simulink model "Mooventure2016_Rev5"  (Simulink 7.7)
settings: Solver=FixedStepDiscrete  StartTime=0.0  StopTime=10  RelTol=1e-3
PreLoadFcn:
  | try, eval([bdroot '_setup']); catch, eval('model_setup', ''); end
InitFcn:
  | try, eval([bdroot '_setup']); catch, eval('model_setup', ''); end
undefined symbols (not defined in the file): ECM, H1, motohawk_build_version, motohawk_trunc_name, motohawk_vardec_config_group, motohawk_vardec_path, xD
libraries: MotoHawk_lib x976, motohawk_control_primitives_lib x41, simulink x27, motohawk_annotations_lib x3
(part 3 of 16)

== system Mooventure2016_Rev5/Foreground/Inputs/ABS ==
  Bus Creator : BusCreator
  Bus Creator1 : BusCreator  Inputs=5
  Bus Creator2 : BusCreator  Inputs=2
  Bus Creator3 : BusCreator  Inputs=3
  Read CAN Message : MotoHawk_lib/CAN Blocks/Read CAN Message  nam=['CAN_' num2str(1)]  bus=-2  msg=CANRx_ABS_217  queue=1  slot=''  valid=off  stale=on  labelwires=on
  Read CAN Message1 : MotoHawk_lib/CAN Blocks/Read CAN Message  nam=['CAN_' num2str(1)]  bus=-2  msg=CANRx_ABS_4B0  queue=1  slot=''  valid=off  stale=on  labelwires=on
  Read CAN Message2 : MotoHawk_lib/CAN Blocks/Read CAN Message  nam=['CAN_' num2str(1)]  bus=-2  msg=CANRx_ABS_417  queue=1  slot=''  valid=off  stale=on  labelwires=on
  motohawk_override_abs1 : MotoHawk_lib/Calibration & Probing Blocks/motohawk_override_abs  SystemSampleTime=-1  parent_name='RT_Wheel_Rolling_Count_Ovr'  parent_val=0  show_more=off  name_source=Use Parameter  parent_read_level=1  parent_override_level=1  view_as=Number  enum_struct={'Disabled', 'Enabled'}  use_help_units=off  parent_help=''  parent_units=''  use_min_max=off  parent_min=-inf  parent_max=inf  use_precision=off  parent_precision=''  parent_gain=1  parent_offset=0  parent_exp=1  use_mototune_group=off  parent_group=motohawk_vardec_path(gcb)
  motohawk_override_abs10 : MotoHawk_lib/Calibration & Probing Blocks/motohawk_override_abs  SystemSampleTime=-1  parent_name='TCS_ENG_EVNT_IN_PROGRESS_Ovr'  parent_val=0  show_more=off  name_source=Use Parameter  parent_read_level=1  parent_override_level=1  view_as=Number  enum_struct={'Disabled', 'Enabled'}  use_help_units=off  parent_help=''  parent_units=''  use_min_max=off  parent_min=-inf  parent_max=inf  use_precision=off  parent_precision=''  parent_gain=1  parent_offset=0  parent_exp=1  use_mototune_group=off  parent_group=motohawk_vardec_path(gcb)
  motohawk_override_abs11 : MotoHawk_lib/Calibration & Probing Blocks/motohawk_override_abs  SystemSampleTime=-1  parent_name='ABS_417_AgeCount_Ovr'  parent_val=0  show_more=off  name_source=Use Parameter  parent_read_level=1  parent_override_level=1  view_as=Number  enum_struct={'Disabled', 'Enabled'}  use_help_units=off  parent_help=''  parent_units=''  use_min_max=off  parent_min=-inf  parent_max=inf  use_precision=off  parent_precision=''  parent_gain=1  parent_offset=0  parent_exp=1  use_mototune_group=off  parent_group=motohawk_vardec_path(gcb)
  motohawk_override_abs2 : MotoHawk_lib/Calibration & Probing Blocks/motohawk_override_abs  SystemSampleTime=-1  parent_name='Wheel_Rolling_Timestamp_Ovr'  parent_val=0  show_more=off  name_source=Use Parameter  parent_read_level=1  parent_override_level=1  view_as=Number  enum_struct={'Disabled', 'Enabled'}  use_help_units=off  parent_help=''  parent_units=''  use_min_max=off  parent_min=-inf  parent_max=inf  use_precision=off  parent_precision=''  parent_gain=1  parent_offset=0  parent_exp=1  use_mototune_group=off  parent_group=motohawk_vardec_path(gcb)
  motohawk_override_abs3 : MotoHawk_lib/Calibration & Probing Blocks/motohawk_override_abs  SystemSampleTime=-1  parent_name='ABS_217_AgeCount_Ovr'  parent_val=0  show_more=off  name_source=Use Parameter  parent_read_level=1  parent_override_level=1  view_as=Number  enum_struct={'Disabled', 'Enabled'}  use_help_units=off  parent_help=''  parent_units=''  use_min_max=off  parent_min=-inf  parent_max=inf  use_precision=off  parent_precision=''  parent_gain=1  parent_offset=0  parent_exp=1  use_mototune_group=off  parent_group=motohawk_vardec_path(gcb)
  motohawk_override_abs4 : MotoHawk_lib/Calibration & Probing Blocks/motohawk_override_abs  SystemSampleTime=-1  parent_name='Front_right_whl_speed_Ovr'  parent_val=0  show_more=off  name_source=Use Parameter  parent_read_level=1  parent_override_level=1  view_as=Number  enum_struct={'Disabled', 'Enabled'}  use_help_units=off  parent_help=''  parent_units=''  use_min_max=off  parent_min=-inf  parent_max=inf  use_precision=off  parent_precision=''  parent_gain=1  parent_offset=0  parent_exp=1  use_mototune_group=off  parent_group=motohawk_vardec_path(gcb)
  motohawk_override_abs5 : MotoHawk_lib/Calibration & Probing Blocks/motohawk_override_abs  SystemSampleTime=-1  parent_name='Rear_left_whl_speed_Ovr'  parent_val=0  show_more=off  name_source=Use Parameter  parent_read_level=1  parent_override_level=1  view_as=Number  enum_struct={'Disabled', 'Enabled'}  use_help_units=off  parent_help=''  parent_units=''  use_min_max=off  parent_min=-inf  parent_max=inf  use_precision=off  parent_precision=''  parent_gain=1  parent_offset=0  parent_exp=1  use_mototune_group=off  parent_group=motohawk_vardec_path(gcb)
  motohawk_override_abs6 : MotoHawk_lib/Calibration & Probing Blocks/motohawk_override_abs  SystemSampleTime=-1  parent_name='ABS_4B0_AgeCount_Ovr'  parent_val=0  show_more=off  name_source=Use Parameter  parent_read_level=1  parent_override_level=1  view_as=Number  enum_struct={'Disabled', 'Enabled'}  use_help_units=off  parent_help=''  parent_units=''  use_min_max=off  parent_min=-inf  parent_max=inf  use_precision=off  parent_precision=''  parent_gain=1  parent_offset=0  parent_exp=1  use_mototune_group=off  parent_group=motohawk_vardec_path(gcb)
  motohawk_override_abs7 : MotoHawk_lib/Calibration & Probing Blocks/motohawk_override_abs  SystemSampleTime=-1  parent_name='LF_Wheel_Rolling_Count_Ovr'  parent_val=0  show_more=off  name_source=Use Parameter  parent_read_level=1  parent_override_level=1  view_as=Number  enum_struct={'Disabled', 'Enabled'}  use_help_units=off  parent_help=''  parent_units=''  use_min_max=off  parent_min=-inf  parent_max=inf  use_precision=off  parent_precision=''  parent_gain=1  parent_offset=0  parent_exp=1  use_mototune_group=off  parent_group=motohawk_vardec_path(gcb)
  motohawk_override_abs8 : MotoHawk_lib/Calibration & Probing Blocks/motohawk_override_abs  SystemSampleTime=-1  parent_name='Front_left_whl_speed_Ovr'  parent_val=0  show_more=off  name_source=Use Parameter  parent_read_level=1  parent_override_level=1  view_as=Number  enum_struct={'Disabled', 'Enabled'}  use_help_units=off  parent_help=''  parent_units=''  use_min_max=off  parent_min=-inf  parent_max=inf  use_precision=off  parent_precision=''  parent_gain=1  parent_offset=0  parent_exp=1  use_mototune_group=off  parent_group=motohawk_vardec_path(gcb)
  motohawk_override_abs9 : MotoHawk_lib/Calibration & Probing Blocks/motohawk_override_abs  SystemSampleTime=-1  parent_name='Rear_right_whl_speed_Ovr'  parent_val=0  show_more=off  name_source=Use Parameter  parent_read_level=1  parent_override_level=1  view_as=Number  enum_struct={'Disabled', 'Enabled'}  use_help_units=off  parent_help=''  parent_units=''  use_min_max=off  parent_min=-inf  parent_max=inf  use_precision=off  parent_precision=''  parent_gain=1  parent_offset=0  parent_exp=1  use_mototune_group=off  parent_group=motohawk_vardec_path(gcb)
  motohawk_probe1 : MotoHawk_lib/Calibration & Probing Blocks/motohawk_probe  nam='RT_Wheel_Rolling_Count_Prb'  show_more=off  name_source=Use Parameter  read_level=1  view_as=Number  enum_struct={'Disabled', 'Enabled'}  vector_style=Wide Row  use_help_units=off  help=''  units=''  use_header_enum=off  row_header_enum={}  col_header_enum={}  use_precision=off  precision=''  gain=1  offset=0  exp=1  use_mototune_group=off  mototune_group=motohawk_vardec_path(gcb)
  motohawk_probe10 : MotoHawk_lib/Calibration & Probing Blocks/motohawk_probe  nam='TCS_ENG_EVNT_IN_PROGRESS_Prb'  show_more=off  name_source=Use Parameter  read_level=1  view_as=Number  enum_struct={'Disabled', 'Enabled'}  vector_style=Wide Row  use_help_units=off  help=''  units=''  use_header_enum=off  row_header_enum={}  col_header_enum={}  use_precision=off  precision=''  gain=1  offset=0  exp=1  use_mototune_group=off  mototune_group=motohawk_vardec_path(gcb)
  motohawk_probe11 : MotoHawk_lib/Calibration & Probing Blocks/motohawk_probe  nam='ABS_417_AgeCount_Prb'  show_more=off  name_source=Use Parameter  read_level=1  view_as=Number  enum_struct={'Disabled', 'Enabled'}  vector_style=Wide Row  use_help_units=off  help=''  units=''  use_header_enum=off  row_header_enum={}  col_header_enum={}  use_precision=off  precision=''  gain=1  offset=0  exp=1  use_mototune_group=off  mototune_group=motohawk_vardec_path(gcb)
  motohawk_probe2 : MotoHawk_lib/Calibration & Probing Blocks/motohawk_probe  nam='Wheel_Rolling_Timestamp_Prb'  show_more=off  name_source=Use Parameter  read_level=1  view_as=Number  enum_struct={'Disabled', 'Enabled'}  vector_style=Wide Row  use_help_units=off  help=''  units=''  use_header_enum=off  row_header_enum={}  col_header_enum={}  use_precision=off  precision=''  gain=1  offset=0  exp=1  use_mototune_group=off  mototune_group=motohawk_vardec_path(gcb)
  motohawk_probe3 : MotoHawk_lib/Calibration & Probing Blocks/motohawk_probe  nam='ABS_217_AgeCount_Prb'  show_more=off  name_source=Use Parameter  read_level=1  view_as=Number  enum_struct={'Disabled', 'Enabled'}  vector_style=Wide Row  use_help_units=off  help=''  units=''  use_header_enum=off  row_header_enum={}  col_header_enum={}  use_precision=off  precision=''  gain=1  offset=0  exp=1  use_mototune_group=off  mototune_group=motohawk_vardec_path(gcb)
  motohawk_probe4 : MotoHawk_lib/Calibration & Probing Blocks/motohawk_probe  nam='Front_right_whl_speed_Prb'  show_more=off  name_source=Use Parameter  read_level=1  view_as=Number  enum_struct={'Disabled', 'Enabled'}  vector_style=Wide Row  use_help_units=off  help=''  units=''  use_header_enum=off  row_header_enum={}  col_header_enum={}  use_precision=off  precision=''  gain=1  offset=0  exp=1  use_mototune_group=off  mototune_group=motohawk_vardec_path(gcb)
  motohawk_probe5 : MotoHawk_lib/Calibration & Probing Blocks/motohawk_probe  nam='Rear_left_whl_speed_Prb'  show_more=off  name_source=Use Parameter  read_level=1  view_as=Number  enum_struct={'Disabled', 'Enabled'}  vector_style=Wide Row  use_help_units=off  help=''  units=''  use_header_enum=off  row_header_enum={}  col_header_enum={}  use_precision=off  precision=''  gain=1  offset=0  exp=1  use_mototune_group=off  mototune_group=motohawk_vardec_path(gcb)
  motohawk_probe6 : MotoHawk_lib/Calibration & Probing Blocks/motohawk_probe  nam='ABS_4B0_AgeCount_Prb'  show_more=off  name_source=Use Parameter  read_level=1  view_as=Number  enum_struct={'Disabled', 'Enabled'}  vector_style=Wide Row  use_help_units=off  help=''  units=''  use_header_enum=off  row_header_enum={}  col_header_enum={}  use_precision=off  precision=''  gain=1  offset=0  exp=1  use_mototune_group=off  mototune_group=motohawk_vardec_path(gcb)
  motohawk_probe7 : MotoHawk_lib/Calibration & Probing Blocks/motohawk_probe  nam='LF_Wheel_Rolling_Count_Prb'  show_more=off  name_source=Use Parameter  read_level=1  view_as=Number  enum_struct={'Disabled', 'Enabled'}  vector_style=Wide Row  use_help_units=off  help=''  units=''  use_header_enum=off  row_header_enum={}  col_header_enum={}  use_precision=off  precision=''  gain=1  offset=0  exp=1  use_mototune_group=off  mototune_group=motohawk_vardec_path(gcb)
  motohawk_probe8 : MotoHawk_lib/Calibration & Probing Blocks/motohawk_probe  nam='Front_left_whl_speed_Prb'  show_more=off  name_source=Use Parameter  read_level=1  view_as=Number  enum_struct={'Disabled', 'Enabled'}  vector_style=Wide Row  use_help_units=off  help=''  units=''  use_header_enum=off  row_header_enum={}  col_header_enum={}  use_precision=off  precision=''  gain=1  offset=0  exp=1  use_mototune_group=off  mototune_group=motohawk_vardec_path(gcb)
  motohawk_probe9 : MotoHawk_lib/Calibration & Probing Blocks/motohawk_probe  nam='Rear_right_whl_speed_Prb'  show_more=off  name_source=Use Parameter  read_level=1  view_as=Number  enum_struct={'Disabled', 'Enabled'}  vector_style=Wide Row  use_help_units=off  help=''  units=''  use_header_enum=off  row_header_enum={}  col_header_enum={}  use_precision=off  precision=''  gain=1  offset=0  exp=1  use_mototune_group=off  mototune_group=motohawk_vardec_path(gcb)
  Out1 : Outport
  wires:
  Read CAN Message/1 -> motohawk_override_abs3/1, motohawk_probe3/1  "AgeCount"
  Read CAN Message/2 -> motohawk_override_abs7/1, motohawk_probe7/1  "LF_Wheel_Rolling_Count"
  Read CAN Message/3 -> motohawk_override_abs1/1, motohawk_probe1/1  "RT_Wheel_Rolling_Count"
  Read CAN Message/4 -> motohawk_override_abs2/1, motohawk_probe2/1  "Wheel_Rolling_Timestamp"
  motohawk_override_abs3/1 -> Bus Creator/1  "AgeCount 217"
  motohawk_override_abs7/1 -> Bus Creator/2  "LF Wheel Rolling Count"
  motohawk_override_abs1/1 -> Bus Creator/3  "RT Wheel Rolling Count"
  motohawk_override_abs2/1 -> Bus Creator/4  "Wheel Rolling Timestamp"
  Read CAN Message1/2 -> motohawk_override_abs8/1, motohawk_probe8/1  "Front_left_whl_speed"
  Read CAN Message1/3 -> motohawk_override_abs4/1, motohawk_probe4/1  "Front_right_whl_speed"
  Read CAN Message1/4 -> motohawk_override_abs5/1, motohawk_probe5/1  "Rear_left_whl_speed"
  motohawk_override_abs6/1 -> Bus Creator1/1  "AgeCount 4B0"
  motohawk_override_abs8/1 -> Bus Creator1/2  "Front left whl speed"
  motohawk_override_abs4/1 -> Bus Creator1/3  "Front right whl speed"
  motohawk_override_abs5/1 -> Bus Creator1/4  "Rear left whl speed"
  Read CAN Message1/1 -> motohawk_override_abs6/1, motohawk_probe6/1  "AgeCount"
  Read CAN Message1/5 -> motohawk_override_abs9/1, motohawk_probe9/1  "Rear_right_whl_speed"
  motohawk_override_abs9/1 -> Bus Creator1/5  "Rear right whl speed"
  Read CAN Message2/1 -> motohawk_override_abs11/1, motohawk_probe11/1  "AgeCount"
  Read CAN Message2/2 -> motohawk_override_abs10/1, motohawk_probe10/1  "TCS_ENG_EVNT_IN_PROGRESS"
  motohawk_override_abs10/1 -> Bus Creator2/2  "ECS Eng Evnt In Progress"
  motohawk_override_abs11/1 -> Bus Creator2/1  "ABS 417 AgeCount"
  Bus Creator/1 -> Bus Creator3/1  "Tone Ring"
  Bus Creator1/1 -> Bus Creator3/2  "Wheel Speed"
  Bus Creator2/1 -> Bus Creator3/3  "Traction Control"
  Bus Creator3/1 -> Out1/1

== system Mooventure2016_Rev5/Foreground/Inputs/Analog Inputs ==
  note: TODO
  Bus Creator : BusCreator  Inputs=3
  Contactors : Subsystem
  Coolant : Subsystem
  DCDC Converter : Subsystem
  Out1 : Outport
  wires:
  Bus Creator/1 -> Out1/1
  Coolant/1(Out1) -> Bus Creator/1  "Coolant"
  DCDC Converter/1(Out1) -> Bus Creator/2  "DCDC"
  Contactors/1(Out1) -> Bus Creator/3  "Contactors"

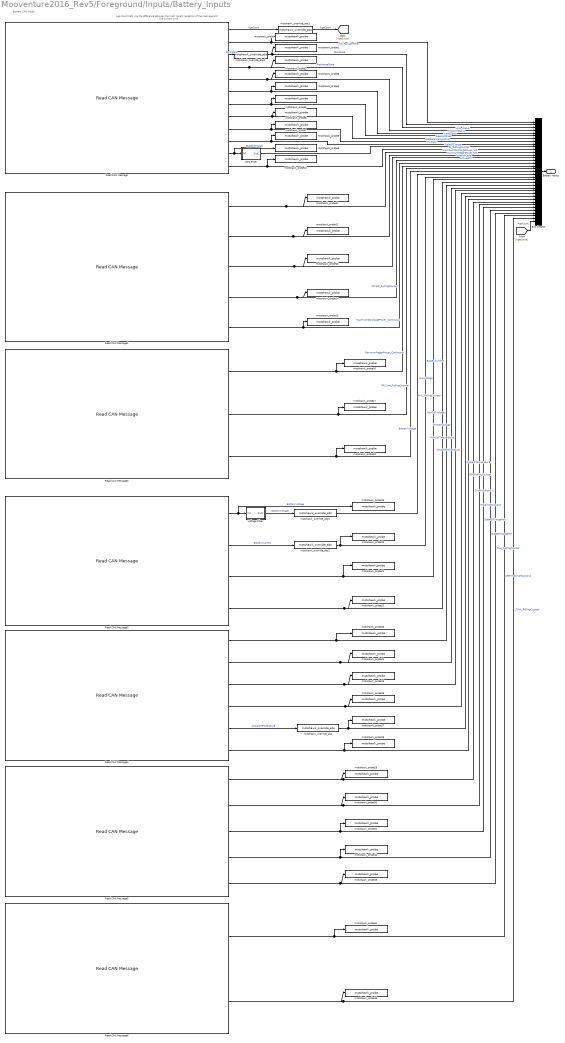
== system Mooventure2016_Rev5/Foreground/Inputs/Battery_Inputs ==
  note: Battery CAN inputs
  note: Age Count tells you the difference between the most recent reception of the message and the current time
  Bus Creator : BusCreator  Inputs=37
  Read CAN Message : MotoHawk_lib/CAN Blocks/Read CAN Message  nam=['CAN_' num2str(3)]  bus=-2  msg=CANRx_BATTERY_2FA  queue=1  slot=''  valid=off  stale=on  labelwires=on
  Read CAN Message1 : MotoHawk_lib/CAN Blocks/Read CAN Message  nam=['CAN_' num2str(3)]  bus=-2  msg=CANRx_BATTERY_2FB  queue=1  slot=''  valid=off  stale=off  labelwires=on
  Read CAN Message2 : MotoHawk_lib/CAN Blocks/Read CAN Message  nam=['CAN_' num2str(3)]  bus=-2  msg=CANRx_Battery_2FC  queue=1  slot=''  valid=off  stale=off  labelwires=on
  Read CAN Message3 : MotoHawk_lib/CAN Blocks/Read CAN Message  nam=['CAN_' num2str(3)]  bus=-2  msg=CANRx_Battery_2FD  queue=1  slot=''  valid=off  stale=off  labelwires=on
  Read CAN Message4 : MotoHawk_lib/CAN Blocks/Read CAN Message  nam=['CAN_' num2str(3)]  bus=-2  msg=CANRx_Battery_2FE  queue=1  slot=''  valid=off  stale=off  labelwires=on
  Read CAN Message5 : MotoHawk_lib/CAN Blocks/Read CAN Message  nam=['CAN_' num2str(3)]  bus=-2  msg=CANRx_Battery_2FF  queue=1  slot=''  valid=off  stale=off  labelwires=on
  Read CAN Message6 : MotoHawk_lib/CAN Blocks/Read CAN Message  nam=['CAN_' num2str(3)]  bus=-2  msg=CANRx_Battery_300  queue=1  slot=''  valid=off  stale=off  labelwires=on
  SOC Filter : Subsystem
  Voltage Filter : Subsystem
  motohawk_override_abs : MotoHawk_lib/Calibration & Probing Blocks/motohawk_override_abs  SystemSampleTime=-1  parent_name='Batt_Coolant_Temp_ovr'  parent_val=0  show_more=off  name_source=Use Parameter  parent_read_level=1  parent_override_level=1  view_as=Number  enum_struct={'Disabled', 'Enabled'}  use_help_units=off  parent_help=''  parent_units=''  use_min_max=off  parent_min=-inf  parent_max=inf  use_precision=off  parent_precision=''  parent_gain=1  parent_offset=0  parent_exp=1  use_mototune_group=off  parent_group=motohawk_vardec_path(gcb)
  motohawk_override_abs2 : MotoHawk_lib/Calibration & Probing Blocks/motohawk_override_abs  SystemSampleTime=-1  parent_name='Batt_Current_ovr'  parent_val=0  show_more=off  name_source=Use Parameter  parent_read_level=1  parent_override_level=1  view_as=Number  enum_struct={'Disabled', 'Enabled'}  use_help_units=off  parent_help=''  parent_units=''  use_min_max=off  parent_min=-inf  parent_max=inf  use_precision=off  parent_precision=''  parent_gain=1  parent_offset=0  parent_exp=1  use_mototune_group=off  parent_group=motohawk_vardec_path(gcb)
  motohawk_override_abs3 : MotoHawk_lib/Calibration & Probing Blocks/motohawk_override_abs  SystemSampleTime=-1  parent_name='Batt_Age_Count_ovr'  parent_val=0  show_more=off  name_source=Use Parameter  parent_read_level=1  parent_override_level=1  view_as=Number  enum_struct={'Disabled', 'Enabled'}  use_help_units=off  parent_help=''  parent_units=''  use_min_max=off  parent_min=-inf  parent_max=inf  use_precision=off  parent_precision=''  parent_gain=1  parent_offset=0  parent_exp=1  use_mototune_group=off  parent_group=motohawk_vardec_path(gcb)
  motohawk_override_abs4 : MotoHawk_lib/Calibration & Probing Blocks/motohawk_override_abs  SystemSampleTime=-1  parent_name='Pack_State_ovr'  parent_val=0  show_more=on  name_source=Use Parameter  parent_read_level=1  parent_override_level=1  view_as=Number  enum_struct={'Disabled', 'Enabled'}  use_help_units=off  parent_help=''  parent_units=''  use_min_max=on  parent_min=0  parent_max=8  use_precision=off  parent_precision=''  parent_gain=1  parent_offset=0  parent_exp=1  use_mototune_group=off  parent_group=motohawk_vardec_path(gcb)
  motohawk_override_abs5 : MotoHawk_lib/Calibration & Probing Blocks/motohawk_override_abs  SystemSampleTime=-1  parent_name='Battery_Voltage_ovr'  parent_val=0  show_more=on  name_source=Use Parameter  parent_read_level=1  parent_override_level=1  view_as=Number  enum_struct={'Disabled', 'Enabled'}  use_help_units=off  parent_help=''  parent_units=''  use_min_max=on  parent_min=0  parent_max=65535  use_precision=off  parent_precision=''  parent_gain=1  parent_offset=0  parent_exp=1  use_mototune_group=off  parent_group=motohawk_vardec_path(gcb)
  motohawk_probe{,1..35} (36 alike) : MotoHawk_lib/Calibration & Probing Blocks/motohawk_probe  nam='Probe'  show_more=on  name_source=Use Input Wire Name  read_level=1  view_as=Number  enum_struct={'Disabled', 'Enabled'}  vector_style=Wide Row  use_help_units=off  help=''  units=''  use_header_enum=off  row_header_enum={}  col_header_enum={}  use_precision=off  precision=''  gain=1  offset=0  exp=1  use_mototune_group=off  mototune_group=motohawk_vardec_path(gcb)
  Battery Inputs : Outport
  wires:
  Read CAN Message/1 -> motohawk_override_abs3/1  "AgeCount"
  Read CAN Message/2 -> Bus Creator/1, motohawk_probe/1  "JCS_PackIdentifier"
  Read CAN Message/4 -> motohawk_probe2/1, Bus Creator/3  "PrechargeState"
  Read CAN Message/5 -> motohawk_probe3/1, Bus Creator/4  "HVIL_Status"
  Read CAN Message/6 -> Bus Creator/5, motohawk_probe4/1  "IsolationStatus"
  Read CAN Message/7 -> Bus Creator/6, motohawk_probe5/1  "WakeSignal"
  Read CAN Message/8 -> Bus Creator/7, motohawk_probe6/1  "SleepInhibited"
  Read CAN Message/9 -> Bus Creator/8, motohawk_probe7/1  "CellBalanceingActive"
  Read CAN Message/10 -> Bus Creator/9, motohawk_probe8/1  "MILState"
  Read CAN Message/12 -> Bus Creator/11, motohawk_probe10/1  "PS_RollingCounter"
  Read CAN Message1/1 -> Bus Creator/12, motohawk_probe11/1  "MaximumDischargePower_10s"
  Read CAN Message1/2 -> Bus Creator/13, motohawk_probe12/1  "MaximumRegenPower_10s"
  Read CAN Message1/3 -> Bus Creator/14, motohawk_probe13/1  "IsolationLevel"
  Read CAN Message1/4 -> Bus Creator/15, motohawk_probe14/1  "ActiveDTC"
  Read CAN Message1/5 -> Bus Creator/16, motohawk_probe15/1  "PPL10s_RollingCounter"
  Read CAN Message2/1 -> Bus Creator/17, motohawk_probe16/1  "MaximumDischargePower_Continuous"
  Read CAN Message2/2 -> Bus Creator/18, motohawk_probe17/1  "MaximumRegenPower_Continuous"
  Read CAN Message2/3 -> Bus Creator/19, motohawk_probe18/1  "PPLCont_RollingCounter"
  Read CAN Message3/3 -> Bus Creator/22, motohawk_probe21/1  "BusVoltage"
  Read CAN Message3/4 -> Bus Creator/23, motohawk_probe22/1  "PVC_RollingCounter"
  Read CAN Message4/1 -> Bus Creator/24, motohawk_probe23/1  "MaxCellVoltage"
  Read CAN Message4/2 -> Bus Creator/25, motohawk_probe24/1  "MinCellVoltage"
  Read CAN Message4/3 -> Bus Creator/26, motohawk_probe25/1  "MaxCellTemperature"
  Read CAN Message4/4 -> Bus Creator/27, motohawk_probe26/1  "MinCellTemperature"
  Read CAN Message4/5 -> motohawk_override_abs/1  "CoolantTemperature"
  Read CAN Message4/6 -> Bus Creator/29, motohawk_probe28/1  "DPI_RollingCounter"
  Read CAN Message5/2 -> Bus Creator/31, motohawk_probe30/1  "TripAmpHoursOut"
  Read CAN Message5/3 -> Bus Creator/32, motohawk_probe31/1  "StateOfChargeMax"
  Read CAN Message5/4 -> Bus Creator/33, motohawk_probe32/1  "StateOfChargeMin"
  Read CAN Message5/5 -> Bus Creator/34, motohawk_probe33/1  "TAH_RollingCounter"
  Read CAN Message6/1 -> Bus Creator/35, motohawk_probe34/1  "LifeTimeAmpHoursOut"
  Read CAN Message6/2 -> Bus Creator/36, motohawk_probe35/1  "LTAHI_RollingCounter"
  Bus Creator/1 -> Battery Inputs/1
  motohawk_override_abs/1 -> Bus Creator/28, motohawk_probe27/1  "CoolantTemperature"
  motohawk_override_abs2/1 -> Bus Creator/21, motohawk_probe20/1  "BatteryCurrent"
  motohawk_override_abs3/1 -> [AgeCount]  "AgeCount"
  Read CAN Message/3 -> motohawk_override_abs4/1  "PackState"
  motohawk_override_abs4/1 -> Bus Creator/2, motohawk_probe1/1  "PackState"
  motohawk_override_abs5/1 -> Bus Creator/20  "BatteryVoltage"
  Read CAN Message5/1 -> Bus Creator/30, motohawk_probe29/1  "TripAmpHoursIn"
  [AgeCount] -> Bus Creator/37  "AgeCount"
  Read CAN Message3/2 -> motohawk_override_abs2/1  "BatteryCurrent"
  Read CAN Message3/1 -> Voltage Filter/1(In1), motohawk_probe19/1  "BatteryVoltage"
  Voltage Filter/1(Out1) -> motohawk_override_abs5/1  "BatteryVoltage"
  SOC Filter/1(Out1) -> Bus Creator/10  "StateOfCharge"
  Read CAN Message/11 -> SOC Filter/1(In1), motohawk_probe9/1  "StateOfCharge"

== system Mooventure2016_Rev5/Foreground/Inputs/CAN Gateway In ==
  Bus Creator : BusCreator  Inputs=2
  Read CAN Message3 : MotoHawk_lib/CAN Blocks/Read CAN Message  nam=['CAN_' num2str(1)]  bus=-2  msg=CANRx_IC_430  queue=1  slot=''  valid=off  stale=off  labelwires=on
  motohawk_override_abs1 : MotoHawk_lib/Calibration & Probing Blocks/motohawk_override_abs  SystemSampleTime=-1  parent_name='AC_Cmd_Ovr'  parent_val=0  show_more=off  name_source=Use Parameter  parent_read_level=1  parent_override_level=1  view_as=Number  enum_struct={'Disabled', 'Enabled'}  use_help_units=off  parent_help=''  parent_units=''  use_min_max=off  parent_min=-inf  parent_max=inf  use_precision=off  parent_precision=''  parent_gain=1  parent_offset=0  parent_exp=1  use_mototune_group=off  parent_group=motohawk_vardec_path(gcb)
  motohawk_override_abs2 : MotoHawk_lib/Calibration & Probing Blocks/motohawk_override_abs  SystemSampleTime=-1  parent_name='Defrost_Mode_Ovr'  parent_val=0  show_more=off  name_source=Use Parameter  parent_read_level=1  parent_override_level=1  view_as=Number  enum_struct={'Disabled', 'Enabled'}  use_help_units=off  parent_help=''  parent_units=''  use_min_max=off  parent_min=-inf  parent_max=inf  use_precision=off  parent_precision=''  parent_gain=1  parent_offset=0  parent_exp=1  use_mototune_group=off  parent_group=motohawk_vardec_path(gcb)
  motohawk_probe1 : MotoHawk_lib/Calibration & Probing Blocks/motohawk_probe  nam='AC_Cmd_Prb'  show_more=off  name_source=Use Parameter  read_level=1  view_as=Number  enum_struct={'Disabled', 'Enabled'}  vector_style=Wide Row  use_help_units=off  help=''  units=''  use_header_enum=off  row_header_enum={}  col_header_enum={}  use_precision=off  precision=''  gain=1  offset=0  exp=1  use_mototune_group=off  mototune_group=motohawk_vardec_path(gcb)
  motohawk_probe2 : MotoHawk_lib/Calibration & Probing Blocks/motohawk_probe  nam='Defrost_Mode_Prb'  show_more=off  name_source=Use Parameter  read_level=1  view_as=Number  enum_struct={'Disabled', 'Enabled'}  vector_style=Wide Row  use_help_units=off  help=''  units=''  use_header_enum=off  row_header_enum={}  col_header_enum={}  use_precision=off  precision=''  gain=1  offset=0  exp=1  use_mototune_group=off  mototune_group=motohawk_vardec_path(gcb)
  Out1 : Outport
  wires:
  Read CAN Message3/1 -> motohawk_override_abs2/1, motohawk_probe2/1  "HEV_CC_Defrost_Mode"
  Read CAN Message3/2 -> motohawk_override_abs1/1, motohawk_probe1/1  "AC_Engaged_CMD"
  motohawk_override_abs2/1 -> Bus Creator/1  "Defrost"
  motohawk_override_abs1/1 -> Bus Creator/2  "AC_Command"
  Bus Creator/1 -> Out1/1

== system Mooventure2016_Rev5/Foreground/Inputs/Charger Param ==
  Bus Creator : BusCreator  Inputs=2
  motohawk_calibration : MotoHawk_lib/Calibration & Probing Blocks/motohawk_calibration  nam='MaxVoltageCal'  val=383.3  storage=Calibration  show_more=off  name_source=Use Parameter  data_type=Inherit from 'Default Value'  read_level=1  write_level=1  ovr_cals=on  view_as=Number  enum_struct={'Disabled', 'Enabled'}  vector_style=Wide Row  use_help_units=off  help=''  units=''  use_header_enum=off  row_header_enum={}  col_header_enum={}  use_min_max=off  min_val=-inf  max_val=inf  use_precision=off  precision=''  gain=1  offset=0  exp=1  use_mototune_group=off  mototune_group=motohawk_vardec_path(gcb)
  motohawk_calibration1 : MotoHawk_lib/Calibration & Probing Blocks/motohawk_calibration  nam='MaxAmpCal'  val=16  storage=Calibration  show_more=off  name_source=Use Parameter  data_type=Inherit from 'Default Value'  read_level=1  write_level=1  ovr_cals=on  view_as=Number  enum_struct={'Disabled', 'Enabled'}  vector_style=Wide Row  use_help_units=off  help=''  units=''  use_header_enum=off  row_header_enum={}  col_header_enum={}  use_min_max=off  min_val=-inf  max_val=inf  use_precision=off  precision=''  gain=1  offset=0  exp=1  use_mototune_group=off  mototune_group=motohawk_vardec_path(gcb)
  Out1 : Outport
  wires:
  motohawk_calibration1/1 -> Bus Creator/2  "MaxAmp"
  motohawk_calibration/1 -> Bus Creator/1  "MaxVoltage"
  Bus Creator/1 -> Out1/1

== system Mooventure2016_Rev5/Foreground/Inputs/Cruise Control ==
  Bus Creator : BusCreator  Inputs=6
  Button Delay 1 : Subsystem
  Button Delay 2 : Subsystem
  Button Delay 3 : Subsystem
  Button Delay 4 : Subsystem
  Button Delay 5 : Subsystem
  Chart : Stateflow chart  TreatAsAtomicUnit=on
  Compare To Constant : simulink/Logic and Bit Operations/Compare To Constant  SystemSampleTime=-1  relop===  const=1  LogicOutDataTypeMode=boolean
  Compare To Constant1 : simulink/Logic and Bit Operations/Compare To Constant  SystemSampleTime=-1  relop===  const=2  LogicOutDataTypeMode=boolean
  Compare To Constant2 : simulink/Logic and Bit Operations/Compare To Constant  SystemSampleTime=-1  relop===  const=3  LogicOutDataTypeMode=boolean
  Compare To Constant3 : simulink/Logic and Bit Operations/Compare To Constant  SystemSampleTime=-1  relop===  const=4  LogicOutDataTypeMode=boolean
  Compare To Constant4 : simulink/Logic and Bit Operations/Compare To Constant  SystemSampleTime=-1  relop===  const=5  LogicOutDataTypeMode=boolean
  Data Type Conversion : DataTypeConversion  OutDataTypeStr=double
  Terminator : Terminator
  motohawk_ain4 : MotoHawk_lib/Analog I//O Blocks/motohawk_ain  res_name=[]  text_resource=AN23  code_resource=NONE  val_resource=-1  target=ECM-5554-112-0904-xD  resource_enum_str=(None)=-1,AN24=1,AN25=2,AN26=3,AN27=4,AN28=5,AN29=6,AN30=7,AN31=8,AN32=9,AN33=10,ECUP=11,ESTOP=12,DRVP=13,XDRP=14,XDRP_B=15,AN1=16,AN2=17,AN3=18,AN4=19,AN5=20,AN6=21,AN7=22,AN8=23,AN9=24,AN10=25,AN11=26,AN12=27,AN13=28,AN14=29,AN15=30,AN16=31,AN17=32,AN18=33,AN19=34,AN20=35,AN21=36,AN22=37,AN23=38,O2A=39,O2B=40,O2C=41,O2D=42  altref=5V Reference  typ=uint16  num_adc_bits=12  use_stat=on  use_vardec=on  nam='Cruise_Control'  read_level=1  write_level=1  group='I/O Pins | Inputs Config'
  motohawk_calibration : MotoHawk_lib/Calibration & Probing Blocks/motohawk_calibration  nam='Off'  val=4092  storage=Calibration  show_more=off  name_source=Use Parameter  data_type=Inherit from 'Default Value'  read_level=1  write_level=1  ovr_cals=on  view_as=Number  enum_struct={'Disabled', 'Enabled'}  vector_style=Wide Row  use_help_units=off  help=''  units=''  use_header_enum=off  row_header_enum={}  col_header_enum={}  use_min_max=off  min_val=-inf  max_val=inf  use_precision=off  precision=''  gain=1  offset=0  exp=1  use_mototune_group=off  mototune_group=motohawk_vardec_path(gcb)
  motohawk_calibration1 : MotoHawk_lib/Calibration & Probing Blocks/motohawk_calibration  nam='SetMinus'  val=4085  storage=Calibration  show_more=off  name_source=Use Parameter  data_type=Inherit from 'Default Value'  read_level=1  write_level=1  ovr_cals=on  view_as=Number  enum_struct={'Disabled', 'Enabled'}  vector_style=Wide Row  use_help_units=off  help=''  units=''  use_header_enum=off  row_header_enum={}  col_header_enum={}  use_min_max=off  min_val=-inf  max_val=inf  use_precision=off  precision=''  gain=1  offset=0  exp=1  use_mototune_group=off  mototune_group=motohawk_vardec_path(gcb)
  motohawk_calibration2 : MotoHawk_lib/Calibration & Probing Blocks/motohawk_calibration  nam='SetPlus'  val=4081  storage=Calibration  show_more=off  name_source=Use Parameter  data_type=Inherit from 'Default Value'  read_level=1  write_level=1  ovr_cals=on  view_as=Number  enum_struct={'Disabled', 'Enabled'}  vector_style=Wide Row  use_help_units=off  help=''  units=''  use_header_enum=off  row_header_enum={}  col_header_enum={}  use_min_max=off  min_val=-inf  max_val=inf  use_precision=off  precision=''  gain=1  offset=0  exp=1  use_mototune_group=off  mototune_group=motohawk_vardec_path(gcb)
  motohawk_calibration3 : MotoHawk_lib/Calibration & Probing Blocks/motohawk_calibration  nam='RSM'  val=4071  storage=Calibration  show_more=off  name_source=Use Parameter  data_type=Inherit from 'Default Value'  read_level=1  write_level=1  ovr_cals=on  view_as=Number  enum_struct={'Disabled', 'Enabled'}  vector_style=Wide Row  use_help_units=off  help=''  units=''  use_header_enum=off  row_header_enum={}  col_header_enum={}  use_min_max=off  min_val=-inf  max_val=inf  use_precision=off  precision=''  gain=1  offset=0  exp=1  use_mototune_group=off  mototune_group=motohawk_vardec_path(gcb)
  motohawk_calibration4 : MotoHawk_lib/Calibration & Probing Blocks/motohawk_calibration  nam='ON'  val=4053  storage=Calibration  show_more=off  name_source=Use Parameter  data_type=Inherit from 'Default Value'  read_level=1  write_level=1  ovr_cals=on  view_as=Number  enum_struct={'Disabled', 'Enabled'}  vector_style=Wide Row  use_help_units=off  help=''  units=''  use_header_enum=off  row_header_enum={}  col_header_enum={}  use_min_max=off  min_val=-inf  max_val=inf  use_precision=off  precision=''  gain=1  offset=0  exp=1  use_mototune_group=off  mototune_group=motohawk_vardec_path(gcb)
  motohawk_calibration5 : MotoHawk_lib/Calibration & Probing Blocks/motohawk_calibration  nam='HYST'  val=3  storage=Calibration  show_more=off  name_source=Use Parameter  data_type=Inherit from 'Default Value'  read_level=1  write_level=1  ovr_cals=on  view_as=Number  enum_struct={'Disabled', 'Enabled'}  vector_style=Wide Row  use_help_units=off  help=''  units=''  use_header_enum=off  row_header_enum={}  col_header_enum={}  use_min_max=off  min_val=-inf  max_val=inf  use_precision=off  precision=''  gain=1  offset=0  exp=1  use_mototune_group=off  mototune_group=motohawk_vardec_path(gcb)
  motohawk_calibration6 : MotoHawk_lib/Calibration & Probing Blocks/motohawk_calibration  nam='DefaultLevel'  val=4012  storage=Calibration  show_more=off  name_source=Use Parameter  data_type=Inherit from 'Default Value'  read_level=1  write_level=1  ovr_cals=on  view_as=Number  enum_struct={'Disabled', 'Enabled'}  vector_style=Wide Row  use_help_units=off  help=''  units=''  use_header_enum=off  row_header_enum={}  col_header_enum={}  use_min_max=off  min_val=-inf  max_val=inf  use_precision=off  precision=''  gain=1  offset=0  exp=1  use_mototune_group=off  mototune_group=motohawk_vardec_path(gcb)
  motohawk_calibration7 : MotoHawk_lib/Calibration & Probing Blocks/motohawk_calibration  nam='Delay'  val=0.08  storage=Calibration  show_more=off  name_source=Use Parameter  data_type=Inherit from 'Default Value'  read_level=1  write_level=1  ovr_cals=on  view_as=Number  enum_struct={'Disabled', 'Enabled'}  vector_style=Wide Row  use_help_units=off  help=''  units=''  use_header_enum=off  row_header_enum={}  col_header_enum={}  use_min_max=off  min_val=-inf  max_val=inf  use_precision=off  precision=''  gain=1  offset=0  exp=1  use_mototune_group=off  mototune_group=motohawk_vardec_path(gcb)
  motohawk_probe : MotoHawk_lib/Calibration & Probing Blocks/motohawk_probe  nam='Cruise_Control_Prb'  show_more=off  name_source=Use Parameter  read_level=1  view_as=Number  enum_struct={'Disabled', 'Enabled'}  vector_style=Wide Row  use_help_units=off  help=''  units=''  use_header_enum=off  row_header_enum={}  col_header_enum={}  use_precision=off  precision=''  gain=1  offset=0  exp=1  use_mototune_group=off  mototune_group=motohawk_vardec_path(gcb)
  motohawk_probe1 : MotoHawk_lib/Calibration & Probing Blocks/motohawk_probe  nam='Cruise_Control_State_Prb'  show_more=off  name_source=Use Parameter  read_level=1  view_as=Number  enum_struct={'Disabled', 'Enabled'}  vector_style=Wide Row  use_help_units=off  help=''  units=''  use_header_enum=off  row_header_enum={}  col_header_enum={}  use_precision=off  precision=''  gain=1  offset=0  exp=1  use_mototune_group=off  mototune_group=motohawk_vardec_path(gcb)
  Out1 : Outport
  wires:
  motohawk_calibration/1 -> Chart/2(Off)
  motohawk_calibration1/1 -> Chart/3(SetMinus)
  motohawk_calibration2/1 -> Chart/4(SetPlus)
  motohawk_calibration3/1 -> Chart/5(RSM)
  motohawk_calibration4/1 -> Chart/6(ON)
  motohawk_calibration5/1 -> Chart/7(HYST)
  Bus Creator/1 -> Out1/1
  motohawk_calibration6/1 -> Chart/8(Default)
  Chart/1(Out) -> Compare To Constant/1, Compare To Constant1/1, Compare To Constant3/1, Compare To Constant4/1, Compare To Constant2/1, motohawk_probe1/1
  Compare To Constant/1 -> Button Delay 1/1(In1)
  Button Delay 1/1(Out1) -> Bus Creator/2  "Off"
  Compare To Constant1/1 -> Button Delay 2/1(In1)
  Compare To Constant2/1 -> Button Delay 3/1(In1)
  Compare To Constant3/1 -> Button Delay 4/1(In1)
  Compare To Constant4/1 -> Button Delay 5/1(In1)
  Button Delay 2/1(Out1) -> Bus Creator/3  "Set-"
  Button Delay 3/1(Out1) -> Bus Creator/4  "Set+"
  Button Delay 4/1(Out1) -> Bus Creator/5  "RSM"
  Button Delay 5/1(Out1) -> Bus Creator/6  "ON"
  motohawk_calibration7/1 -> Button Delay 1/2(Time), Button Delay 2/2(Time), Button Delay 3/2(Time), Button Delay 4/2(Time), Button Delay 5/2(Time)
  Data Type Conversion/1 -> Chart/1(Switch)
  motohawk_ain4/1 -> Bus Creator/1, motohawk_probe/1, Data Type Conversion/1  "Raw Signal"
  motohawk_ain4/2 -> Terminator/1

== system Mooventure2016_Rev5/Foreground/Inputs/Driver Inputs ==
  note: Does some number mapping for ease-of-use later
  note: The digits of the temperature
      | were encoded seperately
  note: 1 - reverse
      | 2 - neutral
      | 3 - drive
  note: NOT IMPLEMENTED FULLY - NEEDS PROBING CAN MESSAGE
  Bus Creator : BusCreator  Inputs=9
  Embedded MATLAB Function : Stateflow chart  TreatAsAtomicUnit=on
  Embedded MATLAB Function1 : Stateflow chart  TreatAsAtomicUnit=on
  Embedded MATLAB Function2 : Stateflow chart  TreatAsAtomicUnit=on
  Read CAN Message1 : MotoHawk_lib/CAN Blocks/Read CAN Message  nam=['CAN_' num2str(3)]  bus=-2  msg=CANRx_TRANSMISSION_510  queue=1  slot=''  valid=off  stale=on  labelwires=on
  Read CAN Message3 : MotoHawk_lib/CAN Blocks/Read CAN Message  nam=['CAN_' num2str(1)]  bus=-2  msg=CANRx_BRAKES_312  queue=1  slot=''  valid=off  stale=on  labelwires=on
  Read CAN Message4 : MotoHawk_lib/CAN Blocks/Read CAN Message  nam=['CAN_' num2str(3)]  bus=-2  msg=CANRx_IC_728  queue=1  slot=''  valid=off  stale=off  labelwires=on
  Read CAN Message6 : MotoHawk_lib/CAN Blocks/Read CAN Message  nam=['CAN_' num2str(2)]  bus=-2  msg=CANRx_CC_3C8  queue=1  slot=''  valid=off  stale=off  labelwires=on
  Terminator2 : Terminator
  motohawk_ain4 : MotoHawk_lib/Analog I//O Blocks/motohawk_ain  res_name=[]  text_resource=AN15  code_resource=NONE  val_resource=-1  target=ECM-5554-112-0904-xD  resource_enum_str=(None)=-1,AN24=1,AN25=2,AN26=3,AN27=4,AN28=5,AN29=6,AN30=7,AN31=8,AN32=9,AN33=10,ECUP=11,ESTOP=12,DRVP=13,XDRP=14,XDRP_B=15,AN1=16,AN2=17,AN3=18,AN4=19,AN5=20,AN6=21,AN7=22,AN8=23,AN9=24,AN10=25,AN11=26,AN12=27,AN13=28,AN14=29,AN15=30,AN16=31,AN17=32,AN18=33,AN19=34,AN20=35,AN21=36,AN22=37,AN23=38,O2A=39,O2B=40,O2C=41,O2D=42  altref=5V Reference  typ=uint16  num_adc_bits=8  use_stat=on  use_vardec=on  nam='Throttle_Position'  read_level=1  write_level=1  group='I/O Pins | Inputs Config'
  motohawk_probe1 : MotoHawk_lib/Calibration & Probing Blocks/motohawk_probe  nam='Brakes_Position_Probe'  show_more=off  name_source=Use Parameter  read_level=1  view_as=Number  enum_struct={'Disabled', 'Enabled'}  vector_style=Wide Row  use_help_units=off  help=''  units=''  use_header_enum=off  row_header_enum={}  col_header_enum={}  use_precision=off  precision=''  gain=1  offset=0  exp=1  use_mototune_group=off  mototune_group=motohawk_vardec_path(gcb)
  motohawk_probe10 : MotoHawk_lib/Calibration & Probing Blocks/motohawk_probe  nam='Passenger_Temp_Prb'  show_more=off  name_source=Use Parameter  read_level=1  view_as=Number  enum_struct={'Disabled', 'Enabled'}  vector_style=Wide Row  use_help_units=off  help=''  units=''  use_header_enum=off  row_header_enum={}  col_header_enum={}  use_precision=off  precision=''  gain=1  offset=0  exp=1  use_mototune_group=off  mototune_group=motohawk_vardec_path(gcb)
  motohawk_probe18 : MotoHawk_lib/Calibration & Probing Blocks/motohawk_probe  nam='Brakes_Age_Count_Probe'  show_more=off  name_source=Use Parameter  read_level=1  view_as=Number  enum_struct={'Disabled', 'Enabled'}  vector_style=Wide Row  use_help_units=off  help=''  units=''  use_header_enum=off  row_header_enum={}  col_header_enum={}  use_precision=off  precision=''  gain=1  offset=0  exp=1  use_mototune_group=off  mototune_group=motohawk_vardec_path(gcb)
  motohawk_probe2 : MotoHawk_lib/Calibration & Probing Blocks/motohawk_probe  nam='Transmission_Age_Count_Probe'  show_more=off  name_source=Use Parameter  read_level=1  view_as=Number  enum_struct={'Disabled', 'Enabled'}  vector_style=Wide Row  use_help_units=off  help=''  units=''  use_header_enum=off  row_header_enum={}  col_header_enum={}  use_precision=off  precision=''  gain=1  offset=0  exp=1  use_mototune_group=off  mototune_group=motohawk_vardec_path(gcb)
  motohawk_probe3 : MotoHawk_lib/Calibration & Probing Blocks/motohawk_probe  nam='Transmission_Position_Probe'  show_more=off  name_source=Use Parameter  read_level=1  view_as=Number  enum_struct={'Disabled', 'Enabled'}  vector_style=Wide Row  use_help_units=off  help=''  units=''  use_header_enum=off  row_header_enum={}  col_header_enum={}  use_precision=off  precision=''  gain=1  offset=0  exp=1  use_mototune_group=off  mototune_group=motohawk_vardec_path(gcb)
  motohawk_probe4 : MotoHawk_lib/Calibration & Probing Blocks/motohawk_probe  nam='Throttle_Position_Prb'  show_more=off  name_source=Use Parameter  read_level=1  view_as=Number  enum_struct={'Disabled', 'Enabled'}  vector_style=Wide Row  use_help_units=off  help=''  units=''  use_header_enum=off  row_header_enum={}  col_header_enum={}  use_precision=off  precision=''  gain=1  offset=0  exp=1  use_mototune_group=off  mototune_group=motohawk_vardec_path(gcb)
  motohawk_probe8 : MotoHawk_lib/Calibration & Probing Blocks/motohawk_probe  nam='Button_Pressed_Prb'  show_more=off  name_source=Use Parameter  read_level=1  view_as=Number  enum_struct={'Disabled', 'Enabled'}  vector_style=Wide Row  use_help_units=off  help=''  units=''  use_header_enum=off  row_header_enum={}  col_header_enum={}  use_precision=off  precision=''  gain=1  offset=0  exp=1  use_mototune_group=off  mototune_group=motohawk_vardec_path(gcb)
  motohawk_probe9 : MotoHawk_lib/Calibration & Probing Blocks/motohawk_probe  nam='Driver_Temp_Prb'  show_more=off  name_source=Use Parameter  read_level=1  view_as=Number  enum_struct={'Disabled', 'Enabled'}  vector_style=Wide Row  use_help_units=off  help=''  units=''  use_header_enum=off  row_header_enum={}  col_header_enum={}  use_precision=off  precision=''  gain=1  offset=0  exp=1  use_mototune_group=off  mototune_group=motohawk_vardec_path(gcb)
  Out1 : Outport
  wires:
  Read CAN Message3/1 -> motohawk_probe18/1, Bus Creator/1  "AgeCount"
  Read CAN Message3/2 -> Bus Creator/2, motohawk_probe1/1  "Brake_Position"
  Read CAN Message1/1 -> Bus Creator/3, motohawk_probe2/1  "AgeCount"
  Read CAN Message1/2 -> Embedded MATLAB Function/1(posIn), motohawk_probe3/1  "Shift_Position"
  Bus Creator/1 -> Out1/1  "Driver _Inputs"
  Embedded MATLAB Function/1(posOut) -> Bus Creator/4  "Shift_Position"
  Read CAN Message4/1 -> motohawk_probe8/1, Bus Creator/6  "Button_Pressed"
  Embedded MATLAB Function/2(ecoModeOut) -> [ecoMode]
  Read CAN Message6/1 -> Embedded MATLAB Function1/1(driver1)  "DRIVER_1"
  Read CAN Message6/2 -> Embedded MATLAB Function1/2(driver10)  "DRIVER_10"
  Read CAN Message6/3 -> Embedded MATLAB Function2/1(passenger1)  "PASSENGER_1"
  Read CAN Message6/4 -> Embedded MATLAB Function2/2(passenger10)  "PASSENGER_10"
  Embedded MATLAB Function1/1(driverTemp) -> motohawk_probe9/1, Bus Creator/8  "driverTemp"
  Embedded MATLAB Function2/1(passengerTemp) -> motohawk_probe10/1, Bus Creator/9  "passengerTemp"
  motohawk_ain4/2 -> Terminator2/1
  motohawk_ain4/1 -> Bus Creator/5, motohawk_probe4/1  "Throttle_Position"
  [ecoMode] -> Bus Creator/7  "ecoMode"

== system Mooventure2016_Rev5/Foreground/Inputs/Eaton Charger ==
  Bus Creator : BusCreator  Inputs=12
  Bus Creator1 : BusCreator  Inputs=2
  Constant : Constant
  Read CAN Message2 : MotoHawk_lib/CAN Blocks/Read CAN Message  nam='CAN_1'  bus=-2  msg=CANRx_EatonCharger_49  queue=1  slot=''  valid=off  stale=on  labelwires=on
  Relational Operator : RelationalOperator  OutDataTypeStr=boolean
  motohawk_data_def4 : MotoHawk_lib/Data Storage Blocks/motohawk_data_def  nam='Eaton_Plugged_In'  container_nam=''  data=0  typ=boolean  struct_nam='MyStruct'  storage=Volatile  outputRef=off  use_vardec=on  window=Display  read_level=1  write_level=1  ovr_cals=on  view_as=Number  enum_struct={'Disabled', 'Enabled'}  vector_style=Wide Row  use_help_units=off  help=''  units=''  use_header_enum=off  row_header_enum=''  col_header_enum=''  use_min_max=off  min_val=-inf  max_val=inf  use_precision=off  precision=''  gain=1  offset=0  exp=1  use_mototune_group=off  mototune_group=motohawk_vardec_path(gcb)  eval_name=MyData  data_stores=motohawk_sfun_data_def_data_stores  struct_instances=motohawk_sfun_data_def_struct_instances  vardecs=motohawk_sfun_data_def_vardecs
  motohawk_data_write : MotoHawk_lib/Data Storage Blocks/motohawk_data_write  source=Lookup By Name  structure=Scalar  operation=Write entire data structure at once  sz_vec=9  sz_row=2  sz_col=9  typ=boolean  nam='Eaton_Plugged_In'  checkNull=on  write_read_only=off  struct_inst_name=''  struct_name='MyStruct'
  motohawk_override_abs{1..9} (9 alike) : MotoHawk_lib/Calibration & Probing Blocks/motohawk_override_abs  SystemSampleTime=-1  parent_name='Batt_SOC_ovr'  parent_val=0  show_more=on  name_source=Use Input Wire Name  parent_read_level=1  parent_override_level=1  view_as=Number  enum_struct={'Disabled', 'Enabled'}  use_help_units=off  parent_help=''  parent_units=''  use_min_max=off  parent_min=-inf  parent_max=inf  use_precision=off  parent_precision=''  parent_gain=1  parent_offset=0  parent_exp=1  use_mototune_group=off  parent_group=motohawk_vardec_path(gcb)
  motohawk_probe{1..2,4,7..10} (7 alike) : MotoHawk_lib/Calibration & Probing Blocks/motohawk_probe  nam='Park_Probe'  show_more=on  name_source=Use Input Wire Name  read_level=1  view_as=Number  enum_struct={'Disabled', 'Enabled'}  vector_style=Wide Row  use_help_units=off  help=''  units=''  use_header_enum=off  row_header_enum={}  col_header_enum={}  use_precision=off  precision=''  gain=1  offset=0  exp=1  use_mototune_group=off  mototune_group=motohawk_vardec_path(gcb)
  motohawk_probe11 : MotoHawk_lib/Calibration & Probing Blocks/motohawk_probe  nam='MessageChecksumInput_Probe'  show_more=on  name_source=Use Parameter  read_level=1  view_as=Number  enum_struct={'Disabled', 'Enabled'}  vector_style=Wide Row  use_help_units=off  help=''  units=''  use_header_enum=off  row_header_enum={}  col_header_enum={}  use_precision=off  precision=''  gain=1  offset=0  exp=1  use_mototune_group=off  mototune_group=motohawk_vardec_path(gcb)
  motohawk_probe3 : MotoHawk_lib/Calibration & Probing Blocks/motohawk_probe  nam='Mains_Current_Draw_Probe'  show_more=on  name_source=Use Parameter  read_level=1  view_as=Number  enum_struct={'Disabled', 'Enabled'}  vector_style=Wide Row  use_help_units=off  help=''  units=''  use_header_enum=off  row_header_enum={}  col_header_enum={}  use_precision=off  precision=''  gain=1  offset=0  exp=1  use_mototune_group=off  mototune_group=motohawk_vardec_path(gcb)
  motohawk_probe5 : MotoHawk_lib/Calibration & Probing Blocks/motohawk_probe  nam='Mains_Voltage_Probe'  show_more=on  name_source=Use Parameter  read_level=1  view_as=Number  enum_struct={'Disabled', 'Enabled'}  vector_style=Wide Row  use_help_units=off  help=''  units=''  use_header_enum=off  row_header_enum={}  col_header_enum={}  use_precision=off  precision=''  gain=1  offset=0  exp=1  use_mototune_group=off  mototune_group=motohawk_vardec_path(gcb)
  motohawk_probe6 : MotoHawk_lib/Calibration & Probing Blocks/motohawk_probe  nam='Eaton_HV_Charger_Temperature_probe'  show_more=on  name_source=Use Parameter  read_level=1  view_as=Number  enum_struct={'Disabled', 'Enabled'}  vector_style=Wide Row  use_help_units=off  help=''  units=''  use_header_enum=off  row_header_enum={}  col_header_enum={}  use_precision=off  precision=''  gain=1  offset=0  exp=1  use_mototune_group=off  mototune_group=motohawk_vardec_path(gcb)
  Eaton Charger : Outport
  wires:
  Read CAN Message2/2 -> motohawk_probe5/1, motohawk_override_abs9/1  "InputVoltage"
  Read CAN Message2/3 -> motohawk_probe1/1, motohawk_override_abs6/1  "OutputVoltage"
  Read CAN Message2/4 -> motohawk_probe2/1, motohawk_override_abs7/1  "InputCurrentLimitMax"
  Read CAN Message2/5 -> motohawk_probe3/1, motohawk_override_abs8/1  "InputCurrent"
  Read CAN Message2/6 -> motohawk_probe4/1, motohawk_override_abs5/1  "OutputCurrent"
  Read CAN Message2/8 -> motohawk_probe7/1, motohawk_override_abs3/1  "IgnitionStatus"
  Read CAN Message2/9 -> motohawk_probe8/1, motohawk_override_abs2/1  "ChargerState"
  Read CAN Message2/10 -> motohawk_probe9/1, motohawk_override_abs1/1  "FaultSeverityIndicator"
  Read CAN Message2/11 -> Bus Creator/10, motohawk_probe10/1  "MessageCounter"
  Read CAN Message2/12 -> Bus Creator/11, motohawk_probe11/1  "MessageChecksum"
  Read CAN Message2/7 -> motohawk_probe6/1, motohawk_override_abs4/1  "Eaton_HV_Charger_Temperature"
  motohawk_override_abs1/1 -> Bus Creator/9  "FaultSeverityIndicator"
  motohawk_override_abs2/1 -> Bus Creator/8, Relational Operator/1  "ChargerState"
  motohawk_override_abs3/1 -> Bus Creator/7  "IgnitionStatus"
  motohawk_override_abs4/1 -> Bus Creator/6  "Eaton_HV_Charger_Temperature"
  motohawk_override_abs5/1 -> Bus Creator/5  "OutputCurrent"
  motohawk_override_abs8/1 -> Bus Creator/4  "InputCurrent"
  motohawk_override_abs7/1 -> Bus Creator/3  "InputCurrentLimitMax"
  motohawk_override_abs6/1 -> Bus Creator/2  "OutputVoltage"
  motohawk_override_abs9/1 -> Bus Creator/1  "InputVoltage"
  Relational Operator/1 -> motohawk_data_write/1, Bus Creator/12  "Eaton_Plugged_In"
  Constant/1 -> Relational Operator/2
  Bus Creator/1 -> Bus Creator1/2  "Eaton_Charger"
  Read CAN Message2/1 -> Bus Creator1/1  "AgeCount"
  Bus Creator1/1 -> Eaton Charger/1  "Eaton_Charger"
